simulink model "PV_MPPT_BOOST1"  (Simulink 8.3)
settings: Solver=ode45  StartTime=0.0  StopTime=0.7  RelTol=1e-3
undefined symbols (not defined in the file or in its folder): ln
libraries: powerlib x12, simulink x1
settings Model: Creator=Birdman  LastModifiedBy=jt  SimulationMode=accelerator
settings OptimizationCC: InitFltsAndDblsToZero=on  EfficientMapNaN2IntZero=off
settings DebuggingCC: SaveWithParameterizedLinksMsg=none  SignalResolutionControl=TryResolveAllWithWarning  FcnCallInpInsideContextMsg=UseLocalSettings  StateNameClashWarn=none
settings HardwareCC: TargetIntDivRoundTo=Zero  TargetEndianess=LittleEndian  TargetHWDeviceType=MATLAB Host  ProdEqTarget=off
settings CodeAppCC: MaxIdLength=128

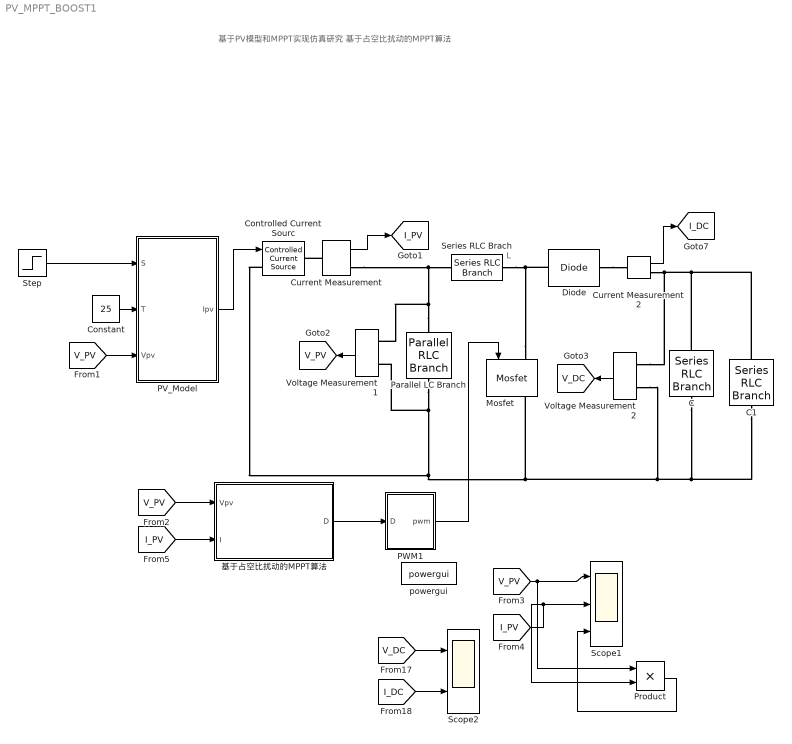
== system PV_MPPT_BOOST1 ==
  note: 基于PV模型和MPPT实现仿真研究
      | 基于占空比扰动的MPPT算法
  note: L
  C : powerlib/Elements/Series RLC Branch  LConnTagsString=__new0  RConnTagsString=__new0  BranchType=C  Resistance=0.5  Inductance=22e-6  SetiL0=off  InitialCurrent=0  Capacitance=10e-6  Setx0=off  InitialVoltage=0  Measurements=None
  C1 : powerlib/Elements/Series RLC Branch  LConnTagsString=__new0  RConnTagsString=__new0  BranchType=R  Resistance=50  Inductance=22e-6  SetiL0=off  InitialCurrent=0  Capacitance=22e-6  Setx0=off  InitialVoltage=0  Measurements=None
  Constant : Constant  Value=25
  Controlled Current Sourc : powerlib/Electrical Sources/Controlled Current Source  Initialize=on  Source_Type=DC  Amplitude=0  Phase=0  Frequency=0  Measurements=None
  Current Measurement : powerlib/Measurements/Current Measurement  PhasorSimulation=off  OutputType=Complex  PSBequivalent=0
  Current Measurement2 : powerlib/Measurements/Current Measurement  PhasorSimulation=off  OutputType=Complex  PSBequivalent=0
  Diode : powerlib/Power Electronics/Diode  Ron=0.001  Lon=0  Vf=0.8  IC=0  UseSnubber=off  Rs=500  Cs=250e-9  Measurements=off
  Mosfet : powerlib/Power Electronics/Mosfet  Ron=0.001  Lon=1e-6  Rd=.001  Vfd=0  IC=0  Rs=1e5  Cs=inf  Measurements=on
  PV_Model : Subsystem  mask{Vm=288, Im=13.88, Voc=354, Isc=14.88, Sref=1000, Tref=25, a=0.0025, b=0.0028, Rs=0.5}
      mask prompts: a "a(A/C)"; b "b(V/C)"
      mask Display: disp('PV_array')
  PWM1 : Subsystem  mask{Ts=1e-6, Fs=2e4}
      mask prompts: Ts "Sample Time"; Fs "Frequency of Tri Wave"
  Parallel LC Branch : powerlib/Elements/Parallel RLC Branch  LConnTagsString=a  RConnTagsString=__new0  BranchType=C  Resistance=1.0  Inductance=1.0  SetiL0=off  InitialCurrent=0  Capacitance=80e-6  Setx0=off  InitialVoltage=0  Measurements=None
  Product : Product
  Scope1 : Scope  NumInputPorts=3
      settings: YMin=358~-4~-1500  YMax=374~1~500
  Scope2 : Scope  NumInputPorts=2
      settings: YMin=407.5~-1  YMax=447.5~15  SaveName=ScopeData3
  Series RLC Brach : powerlib/Elements/Series RLC Branch  LConnTagsString=__new0  RConnTagsString=__new0  BranchType=L  Resistance=0.00  Inductance=9e-3  SetiL0=off  InitialCurrent=0  Capacitance=1.0  Setx0=off  InitialVoltage=0  Measurements=None
  Step : Step  Time=0.3  Before=1000  After=600  SampleTime=0
  Voltage Measurement1 : powerlib/Measurements/Voltage Measurement  PhasorSimulation=off  OutputType=Complex  PSBequivalent=0
  Voltage Measurement2 : powerlib/Measurements/Voltage Measurement  PhasorSimulation=off  OutputType=Complex  PSBequivalent=0
  powergui : powerlib/powergui  SimulationMode=Discrete  SolverType=Tustin  SampleTime=1e-6  frequency=60  SPID=off  DisableSnubberDevices=off  DisableRonSwitches=off  DisableVfSwitches=off  SwTol=0  Interpol=off  DisplayEquations=off  Ts=0  methode=off  frequencyindice=0  Pbase=100e6  ErrMax=1e-4  Iterations=50  UnitsV=kV  UnitsW=MW  FunctionMessages=off  echomessages=off  HookPort=off  EnableUseOfTLC=off  x0status=blocks  RestoreLinks=warning  ResistiveCurrentMeasurement=off  Frange=[0:2:500]  Ylog=off  Xlog=on  ShowGrid=off  save=off  variable=ZData  structure=io  ZoomFFT=off  StartTime=0.0  cycles=3  DisplayStyle=1  fundamental=50  FreqAxis=on  MaxFrequency=2500  frequencyindicesteady=1  RmsSteady=1  display=off
  基于占空比扰动的MPPT算法 : Subsystem  mask{Ts=1e-6, Cp=0.001}
      mask prompts: Ts "Sample Time"; Cp "dD"
  tag scope: I_DC=global, I_PV=global, V_DC=global, V_PV=global
  wires:
  Step/1 -> PV_Model/1(S)
  Constant/1 -> PV_Model/2(T)
  PV_Model/1(Ipv) -> Controlled Current Sourc/1
  Current Measurement/1 -> [I_PV]
  Voltage Measurement1/1 -> [V_PV]
  [V_PV] -> PV_Model/3(Vpv)
  [V_PV] -> 基于占空比扰动的MPPT算法/1(Vpv)
  [I_PV] -> 基于占空比扰动的MPPT算法/2(I)
  Voltage Measurement2/1 -> [V_DC]
  PWM1/1(pwm) -> Mosfet/1
  [V_DC] -> Scope2/1
  [I_DC] -> Scope2/2
  Current Measurement2/1 -> [I_DC]
  基于占空比扰动的MPPT算法/1(D) -> PWM1/1(D)
  [V_PV] -> Product/1, Scope1/1
  [I_PV] -> Product/2, Scope1/2
  Product/1 -> Scope1/3
  connections:
  Parallel LC Branch/LConn1 -- Current Measurement/RConn1 -- Series RLC Brach/LConn1 -- Voltage Measurement1/LConn1
  Mosfet/LConn1 -- Series RLC Brach/RConn1 -- Diode/LConn1
  Current Measurement/LConn1 -- Controlled Current Sourc/RConn1
  Diode/RConn1 -- Current Measurement2/LConn1
  Voltage Measurement2/LConn1 -- C/LConn1 -- C1/LConn1 -- Current Measurement2/RConn1
  C/RConn1 -- C1/RConn1 -- Voltage Measurement2/LConn2 -- Controlled Current Sourc/LConn1 -- Parallel LC Branch/RConn1 -- Voltage Measurement1/LConn2 -- Mosfet/RConn1

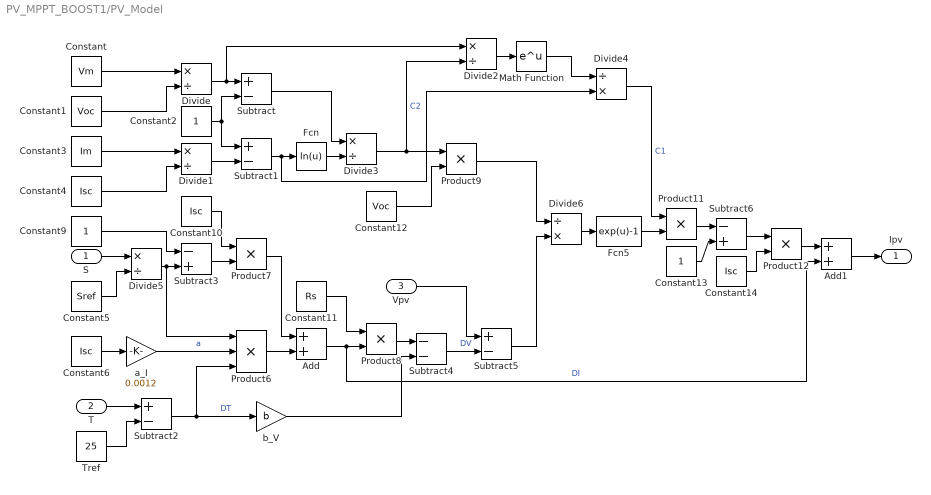
== system PV_MPPT_BOOST1/PV_Model ==
  S : Inport
  T : Inport  Port=2
  Vpv : Inport  Port=3
  Add : Sum
  Add1 : Sum
  Constant : Constant  Value=Vm
  Constant1 : Constant  Value=Voc
  Constant{4,6,10,14} (4 alike) : Constant  Value=Isc
  Constant11 : Constant  Value=Rs
  Constant12 : Constant  Value=Voc
  Constant13 : Constant
  Constant2 : Constant
  Constant3 : Constant  Value=Im
  Constant5 : Constant  Value=Sref
  Constant9 : Constant
  Divide{,1..3,5} (5 alike) : Product  Inputs=*/
  Divide4 : Product  Inputs=/*
  Divide6 : Product  Inputs=/*
  Fcn : Fcn  Expr=ln(u)
  Fcn5 : Fcn  Expr=exp(u)-1
  Math Function : Math  SaturateOnIntegerOverflow=on
  Product{7..9,11..12} (5 alike) : Product  RndMeth=Zero
  Product6 : Product  Inputs=3  RndMeth=Zero
  Subtract{,1..2,5} (4 alike) : Sum  Inputs=+-
  Subtract3 : Sum  Inputs=-+
  Subtract4 : Sum  Inputs=--
  Subtract6 : Sum  Inputs=-+
  Tref : Constant  Value=25
  a_I : Gain  Gain=0.0012
  b_V : Gain  Gain=b
  Ipv : Outport
  wires:
  Constant1/1 -> Divide/2
  Constant/1 -> Divide/1
  Divide/1 -> Subtract/1, Divide2/1
  Constant2/1 -> Subtract/2, Subtract1/1
  Constant4/1 -> Divide1/2
  Constant3/1 -> Divide1/1
  Divide1/1 -> Subtract1/2
  Subtract1/1 -> Divide4/2, Fcn/1
  Subtract/1 -> Divide3/1
  Divide3/1 -> Product9/1, Divide2/2  "C2"
  Divide2/1 -> Math Function/1
  Math Function/1 -> Divide4/1
  Divide4/1 -> Product11/1  "C1"
  T/1 -> Subtract2/1
  Tref/1 -> Subtract2/2
  Subtract2/1 -> Product6/3, b_V/1  "DT"
  S/1 -> Divide5/1
  b_V/1 -> Subtract4/2
  Constant6/1 -> a_I/1
  a_I/1 -> Product6/2  "a"
  Divide5/1 -> Product6/1, Subtract3/2
  Constant9/1 -> Subtract3/1
  Subtract3/1 -> Product7/2
  Constant10/1 -> Product7/1
  Product7/1 -> Add/1
  Product6/1 -> Add/2
  Add/1 -> Product8/2, Add1/2  "DI"
  Constant11/1 -> Product8/1
  Product8/1 -> Subtract4/1
  Subtract4/1 -> Subtract5/2  "DV"
  Constant12/1 -> Product9/2
  Product9/1 -> Divide6/1
  Vpv/1 -> Subtract5/1
  Divide6/1 -> Fcn5/1
  Subtract5/1 -> Divide6/2
  Fcn5/1 -> Product11/2
  Product11/1 -> Subtract6/1
  Constant13/1 -> Subtract6/2
  Subtract6/1 -> Product12/1
  Constant14/1 -> Product12/2
  Product12/1 -> Add1/1
  Add1/1 -> Ipv/1
  Fcn/1 -> Divide3/2
  Constant5/1 -> Divide5/2

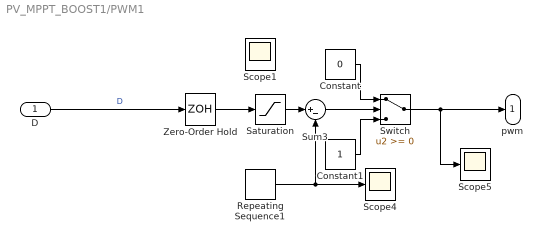
== system PV_MPPT_BOOST1/PWM1 ==
  D : Inport
  Constant : Constant  Value=0
  Constant1 : Constant
  Repeating Sequence1 : simulink/Sources/Repeating Sequence  rep_seq_t=[0 1/Fs/2 1/Fs]  rep_seq_y=[0 1 0]
  Saturation : Saturate  UpperLimit=0.6  LowerLimit=0.5
  Scope1 : Scope
      settings: YMin=0  YMax=3.25  SaveName=ScopeData7
  Scope4 : Scope
      settings: YMin=0.03825  YMax=0.0425  SaveName=ScopeData4
  Scope5 : Scope
      settings: YMin=0.95  YMax=1.05  SaveName=ScopeData5
  Sum3 : Sum  Inputs=|+-
  Switch : Switch
  Zero-Order Hold : ZeroOrderHold  SampleTime=Ts
  pwm : Outport
  wires:
  Saturation/1 -> Sum3/1
  Repeating Sequence1/1 -> Sum3/2, Scope4/1
  Sum3/1 -> Switch/2
  Constant1/1 -> Switch/3
  Constant/1 -> Switch/1
  Switch/1 -> Scope5/1, pwm/1
  Zero-Order Hold/1 -> Saturation/1
  D/1 -> Zero-Order Hold/1  "D"

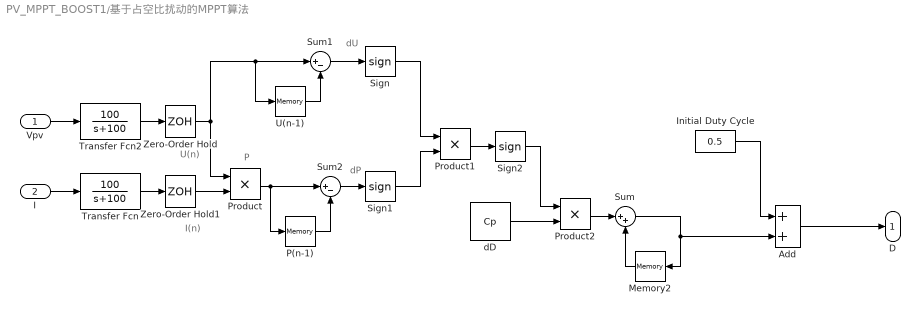
== system PV_MPPT_BOOST1/基于占空比扰动的MPPT算法 ==
  note: U(n)
  note: I(n)
  note: P
  note: dU
  note: dP
  Vpv : Inport
  I : Inport  Port=2
  Add : Sum
  Initial Duty Cycle : Constant  Value=0.5
  Memory2 : Memory
  P(n-1) : Memory  X0=140.538
  Product : Product  RndMeth=Zero
  Product1 : Product  RndMeth=Zero
  Product2 : Product  RndMeth=Zero
  Sign : Signum
  Sign1 : Signum
  Sign2 : Signum
  Sum : Sum  Inputs=|++
  Sum1 : Sum  Inputs=|+-
  Sum2 : Sum  Inputs=|+-
  Transfer Fcn : TransferFcn  Numerator=[100]  Denominator=[1 100]
  Transfer Fcn2 : TransferFcn  Numerator=[100]  Denominator=[1 100]
  U(n-1) : Memory  X0=17.7
  Zero-Order Hold : ZeroOrderHold  SampleTime=Ts
  Zero-Order Hold1 : ZeroOrderHold  SampleTime=Ts
  dD : Constant  Value=Cp
  D : Outport
  wires:
  Sum1/1 -> Sign/1
  U(n-1)/1 -> Sum1/2
  Product/1 -> Sum2/1, P(n-1)/1
  Sum2/1 -> Sign1/1
  P(n-1)/1 -> Sum2/2
  Product1/1 -> Sign2/1
  dD/1 -> Product2/2
  Sign2/1 -> Product2/1
  Product2/1 -> Sum/1
  Sum/1 -> Add/2, Memory2/1
  Memory2/1 -> Sum/2
  Zero-Order Hold1/1 -> Product/2
  Zero-Order Hold/1 -> Product/1, Sum1/1, U(n-1)/1
  Vpv/1 -> Transfer Fcn2/1
  I/1 -> Transfer Fcn/1
  Sign/1 -> Product1/1
  Sign1/1 -> Product1/2
  Transfer Fcn2/1 -> Zero-Order Hold/1
  Transfer Fcn/1 -> Zero-Order Hold1/1
  Initial Duty Cycle/1 -> Add/1
  Add/1 -> D/1
